simulink model "twobit"  (R2016b)
settings: Solver=VariableStepAuto  StartTime=0.0  StopTime=1024  RelTol=1e-3
libraries: xbsIndex_r4 x150, casper_library_misc x3, xps_library x1
settings Model: Creator=nivek  LastModifiedBy=nivek

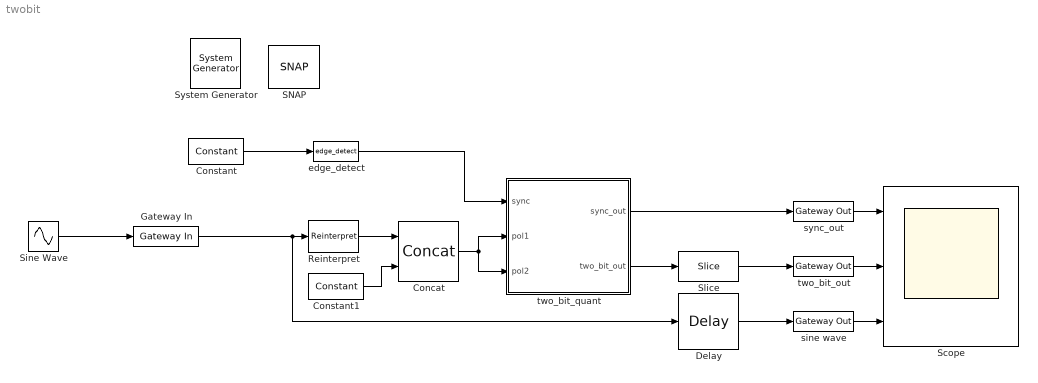
== system twobit ==
  " System Generator" : xbsIndex_r4/ System Generator  Tag=genX  xilinxfamily=kintex7  part=xc7k325t  speed=-3  package=fbg676  synthesis_tool=Vivado  clock_wrapper=Clock Enables  directory=./netlist  proj_type=Vivado  Synth_file=Vivado Synthesis Defaults  Impl_file=Vivado Implementation Defaults  testbench=off  simulink_period=1  sysclk_period=10  dcm_input_clock_period=10  incr_netlist=off  trim_vbits=Everywhere in SubSystem  dbl_ovrd=According to Block Masks  core_generation=According to Block Masks  run_coregen=off  deprecated_control=off  eval_field=0  block_type=sysgen
  Concat : xbsIndex_r4/Concat  num_inputs=2  dbl_ovrd=off  block_type=concat
  Constant : xbsIndex_r4/Constant  const=1.0  gui_display_data_type=Boolean  arith_type=Boolean  n_bits=16  bin_pt=14  preci_type=Single  exp_width=8  frac_width=24  explicit_period=on  period=1  equ=P=C  opselect=C  inp2=PCIN>>17  opr=+  inp1=P  carry=CIN  dbl_ovrd=off  block_type=constant
  Constant1 : xbsIndex_r4/Constant  const=0  gui_display_data_type=Fixed-point  arith_type=Unsigned  n_bits=18  bin_pt=0  preci_type=Single  exp_width=8  frac_width=24  explicit_period=on  period=1  equ=P=C  opselect=C  inp2=PCIN>>17  opr=+  inp1=P  carry=CIN  dbl_ovrd=off  block_type=constant
  Delay : xbsIndex_r4/Delay  rst=off  infoeditControl=Selection of Reset will increase slice count due to use of real FFs and instead of SRLs  en=off  latency=9  reg_retiming=off  dbl_ovrd=off  block_type=delay
  Gateway In : xbsIndex_r4/Gateway In  gui_display_data_type=Fixed-point  arith_type="Signed  (2's comp)"  n_bits=18  bin_pt=17  preci_type=Single  exp_width=8  frac_width=24  rows=1  columns=1  quantization="Round  (unbiased: +/- Inf)"  overflow=Saturate  period=1  UseAsADC=off  ADCChannel='1'  interface=None  automatic_assignment=on  address_offset=hex2dec('00')  intf_name=''  intf_description=''  default_value=0  timing_constraint=None  locs_specified=off  LOCs={}  io_standard={}  inherit_from_input=off  hdl_port=on  dbl_ovrd=off  block_type=gatewayin
  Reinterpret : xbsIndex_r4/Reinterpret  force_arith_type=on  arith_type=Unsigned  force_bin_pt=on  bin_pt=0  block_type=reinterpret
  SNAP : xps_library/Platforms/SNAP  Tag=xps:xsg  hw_sys=SNAP:xc7k160t  clk_src=adc0_clk  clk_rate=250  use_microblaze=off  sample_period=1  synthesis_tool=XST
  Scope : Scope  NumInputPorts=3
  Sine Wave : Sin  SineType=Sample based  Amplitude=0.875  Samples=128  SampleTime=1
  Slice : xbsIndex_r4/Slice  nbits=2  boolean_output=off  mode=Upper Bit Location + Width  bit1=0  base1=MSB of Input  bit0=0  base0=LSB of Input  dbl_ovrd=off  block_type=slice
  edge_detect : casper_library_misc/edge_detect  edge=Rising  polarity=Active High  x_in=[0 0.08 0.08 0.16 0.16 0.24 0.24 0.32 0.32 0.4]  y_in="[-1 -1  1  1  1  1  1  1  1  1]"  x_out=[0.6 0.68 0.68 0.76 0.76 0.84 0.84 0.92 0.92 1]  y_out="[-1 -1  1  1 -1 -1 -1 -1 -1 -1]"
  sine wave : xbsIndex_r4/Gateway Out  inherit_from_input=off  hdl_port=on  rows=1  columns=1  UseAsDAC=off  DACChannel='1'  interface=None  automatic_assignment=on  address_offset=hex2dec('00')  intf_name=''  intf_description=''  timing_constraint=None  locs_specified=off  LOCs={}  io_standard={}  block_type=gatewayout
  sync_out : xbsIndex_r4/Gateway Out  inherit_from_input=off  hdl_port=on  rows=1  columns=1  UseAsDAC=off  DACChannel='1'  interface=None  automatic_assignment=on  address_offset=hex2dec('00')  intf_name=''  intf_description=''  timing_constraint=None  locs_specified=off  LOCs={}  io_standard={}  block_type=gatewayout
  two_bit_out : xbsIndex_r4/Gateway Out  inherit_from_input=off  hdl_port=on  rows=1  columns=1  UseAsDAC=off  DACChannel='1'  interface=None  automatic_assignment=on  address_offset=hex2dec('00')  intf_name=''  intf_description=''  timing_constraint=None  locs_specified=off  LOCs={}  io_standard={}  block_type=gatewayout
  two_bit_quant : Subsystem
  wires:
  two_bit_out/1 -> Scope/2
  sync_out/1 -> Scope/1
  two_bit_quant/1(sync_out) -> sync_out/1
  two_bit_quant/2(two_bit_out) -> Slice/1
  Slice/1 -> two_bit_out/1
  edge_detect/1 -> two_bit_quant/1(sync)
  Constant/1 -> edge_detect/1
  Sine Wave/1 -> Gateway In/1
  sine wave/1 -> Scope/3
  Constant1/1 -> Concat/2
  Concat/1 -> two_bit_quant/3(pol2), two_bit_quant/2(pol1)
  Reinterpret/1 -> Concat/1
  Gateway In/1 -> Delay/1, Reinterpret/1
  Delay/1 -> sine wave/1

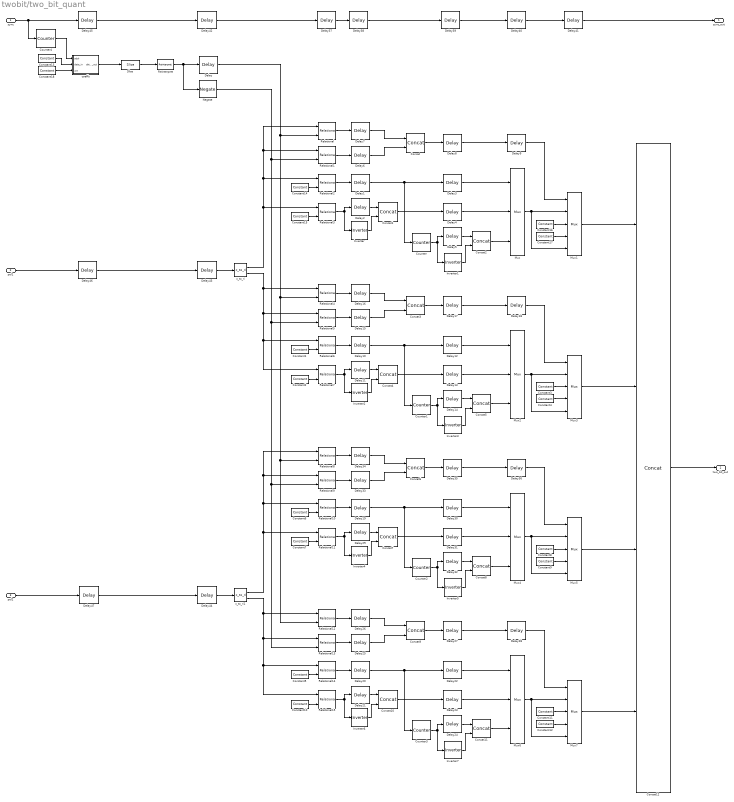
== system twobit/two_bit_quant ==
  sync : Inport
  pol1 : Inport  Port=2
  pol2 : Inport  Port=3
  Concat{,1..11} (12 alike) : xbsIndex_r4/Concat  num_inputs=2  dbl_ovrd=off  block_type=concat
  Concat12 : xbsIndex_r4/Concat  num_inputs=4  dbl_ovrd=off  block_type=concat
  Constant{1..2,5..7,10,14..15} (8 alike) : xbsIndex_r4/Constant  const=0  gui_display_data_type=Fixed-point  arith_type=Signed (2's comp)  n_bits=16  bin_pt=14  preci_type=Single  exp_width=8  frac_width=24  explicit_period=on  period=1  equ=P=C  opselect=C  inp2=PCIN>>17  opr=+  inp1=P  carry=CIN  dbl_ovrd=off  block_type=constant
  Constant{3,8,11,16} (4 alike) : xbsIndex_r4/Constant  const=0  gui_display_data_type=Fixed-point  arith_type=Unsigned  n_bits=2  bin_pt=0  preci_type=Single  exp_width=8  frac_width=24  explicit_period=on  period=1  equ=P=C  opselect=C  inp2=PCIN>>17  opr=+  inp1=P  carry=CIN  dbl_ovrd=off  block_type=constant
  Constant{4,9,12,17} (4 alike) : xbsIndex_r4/Constant  const=3  gui_display_data_type=Fixed-point  arith_type=Unsigned  n_bits=2  bin_pt=0  preci_type=Single  exp_width=8  frac_width=24  explicit_period=on  period=1  equ=P=C  opselect=C  inp2=PCIN>>17  opr=+  inp1=P  carry=CIN  dbl_ovrd=off  block_type=constant
  Constant13 : xbsIndex_r4/Constant  const=0  gui_display_data_type=Fixed-point  arith_type=Signed (2's comp)  n_bits=32  bin_pt=17  preci_type=Single  exp_width=8  frac_width=24  explicit_period=on  period=1  equ=P=C  opselect=C  inp2=PCIN>>17  opr=+  inp1=P  carry=CIN  dbl_ovrd=off  block_type=constant
  Constant18 : xbsIndex_r4/Constant  const=0  gui_display_data_type=Boolean  arith_type=Boolean  n_bits=16  bin_pt=14  preci_type=Single  exp_width=8  frac_width=24  explicit_period=on  period=1  equ=P=C  opselect=C  inp2=PCIN>>17  opr=+  inp1=P  carry=CIN  dbl_ovrd=off  block_type=constant
  Counter{,1..3} (4 alike) : xbsIndex_r4/Counter  cnt_type=Free Running  cnt_to=Inf  operation=Up  start_count=0  cnt_by_val=1  arith_type=Unsigned  n_bits=1  bin_pt=0  load_pin=off  rst=off  en=on  explicit_period=on  period=1  use_behavioral_HDL=off  implementation=Fabric  dbl_ovrd=off  block_type=counter
  Counter4 : xbsIndex_r4/Counter  cnt_type=Free Running  cnt_to=50  operation=Up  start_count=0  cnt_by_val=1  arith_type=Unsigned  n_bits=11  bin_pt=0  load_pin=off  rst=on  en=off  explicit_period=on  period=1  use_behavioral_HDL=off  implementation=Fabric  dbl_ovrd=off  block_type=counter
  Delay{,1..44} (45 alike) : xbsIndex_r4/Delay  rst=off  infoeditControl=Selection of Reset will increase slice count due to use of real FFs and instead of SRLs  en=off  latency=1  reg_retiming=off  dbl_ovrd=off  block_type=delay
  Delay45 : xbsIndex_r4/Delay  rst=off  infoeditControl=Selection of Reset will increase slice count due to use of real FFs and instead of SRLs  en=off  latency=3  reg_retiming=off  dbl_ovrd=off  block_type=delay
  Delay46 : xbsIndex_r4/Delay  rst=off  infoeditControl=Selection of Reset will increase slice count due to use of real FFs and instead of SRLs  en=off  latency=3  reg_retiming=off  dbl_ovrd=off  block_type=delay
  Delay47 : xbsIndex_r4/Delay  rst=off  infoeditControl=Selection of Reset will increase slice count due to use of real FFs and instead of SRLs  en=off  latency=3  reg_retiming=off  dbl_ovrd=off  block_type=delay
  Inverter{,1..7} (8 alike) : xbsIndex_r4/Inverter  en=off  latency=1  dbl_ovrd=off  block_type=inv
  Mux{,2,4,6} (4 alike) : xbsIndex_r4/Mux  inputs=2  en=off  latency=1  precision=Full  arith_type=Unsigned  n_bits=16  bin_pt=14  quantization=Truncate  overflow=Wrap  dbl_ovrd=off  block_type=mux
  Mux{1,3,5,7} (4 alike) : xbsIndex_r4/Mux  inputs=4  en=off  latency=1  precision=Full  arith_type=Unsigned  n_bits=16  bin_pt=14  quantization=Truncate  overflow=Wrap  dbl_ovrd=off  block_type=mux
  Negate : xbsIndex_r4/Negate  precision=User Defined  arith_type="Signed  (2's comp)"  n_bits=18  bin_pt=17  quantization=Truncate  overflow=Wrap  en=off  latency=1  dbl_ovrd=off  block_type=negate
  Reinterpret : xbsIndex_r4/Reinterpret  force_arith_type=on  arith_type="Signed  (2's comp)"  force_bin_pt=on  bin_pt=17  block_type=reinterpret
  Relational{,4,8,12} (4 alike) : xbsIndex_r4/Relational  mode=a>=b  op_type=Bool  en=off  latency=1  dbl_ovrd=off  block_type=relational
  Relational{1,5,9,13} (4 alike) : xbsIndex_r4/Relational  mode=a<=b  op_type=Bool  en=off  latency=1  dbl_ovrd=off  block_type=relational
  Relational{2,6,10,14} (4 alike) : xbsIndex_r4/Relational  mode=a=b  op_type=Bool  en=off  latency=1  dbl_ovrd=off  block_type=relational
  Relational{3,7,11,15} (4 alike) : xbsIndex_r4/Relational  mode=a>b  op_type=Bool  en=off  latency=1  dbl_ovrd=off  block_type=relational
  Slice : xbsIndex_r4/Slice  nbits=18  boolean_output=off  mode=Lower Bit Location + Width  bit1=0  base1=MSB of Input  bit0=0  base0=LSB of Input  dbl_ovrd=off  block_type=slice
  c_to_ri : casper_library_misc/c_to_ri  n_bits=18  bin_pt=17
  c_to_ri1 : casper_library_misc/c_to_ri  n_bits=18  bin_pt=17
  coeffs : Subsystem  Tag=xps:bram  AncestorBlock=xps_library/Memory/shared_bram  mask{arith_type=Unsigned, addr_width=11, data_width=32, reg_prim_output=on, reg_core_output=on, optimization=Minimum_Area, data_bin_pt=0, init_vals=ones(1, 2^11)*65536, sample_rate=1}
      mask prompts: arith_type "Output Data Type"; addr_width "Address width"; data_width "Data Width"; reg_prim_output "Register Primitive Output"; reg_core_output "Register Core Output"; data_bin_pt "Data Binary Point"; init_vals "Initial values (simulation only)"; sample_rate "Sample rate"
      mask init:
      | shared_bram_mask;
      mask TypeOptions arith_type: Unsigned | Signed  (2's comp)
      mask TypeOptions data_width: 8 | 16 | 32 | 64 | 128
      mask TypeOptions optimization: Minimum_Area | Low_Power
  sync_out : Outport
  two_bit_out : Outport  Port=2
  wires:
  Delay41/1 -> sync_out/1
  Delay37/1 -> Delay38/1
  Relational3/1 -> Delay2/1, Inverter/1
  Mux1/1 -> Concat12/1
  Delay5/1 -> Concat2/1
  Constant14/1 -> Relational2/2
  Constant16/1 -> Mux1/3
  Delay38/1 -> Delay39/1
  Delay3/1 -> Mux/1
  Concat2/1 -> Mux/3
  Delay9/1 -> Mux1/1
  Delay8/1 -> Delay9/1
  pol1/1 -> Delay46/1
  sync/1 -> Counter4/1, Delay45/1
  c_to_ri/1 -> Relational3/1, Relational2/1, Relational1/1, Relational/1
  Mux5/1 -> Concat12/3
  Constant15/1 -> Relational3/2
  Delay39/1 -> Delay40/1
  Delay6/1 -> Concat/2
  Mux7/1 -> Concat12/4
  Concat/1 -> Delay8/1
  Delay7/1 -> Concat/1
  Mux/1 -> Mux1/5, Mux1/2
  Inverter/1 -> Concat1/2
  Relational2/1 -> Delay1/1
  Concat12/1 -> two_bit_out/1
  Delay2/1 -> Concat1/1
  Delay1/1 -> Delay3/1, Counter/1
  Delay40/1 -> Delay41/1
  Delay4/1 -> Mux/2
  Relational1/1 -> Delay6/1
  Concat1/1 -> Delay4/1
  Mux3/1 -> Concat12/2
  Relational/1 -> Delay7/1
  Counter/1 -> Inverter1/1, Delay5/1
  Inverter1/1 -> Concat2/2
  Constant17/1 -> Mux1/4
  coeffs/1(data_out) -> Slice/1
  pol2/1 -> Delay47/1
  Delay42/1 -> Delay37/1
  Relational7/1 -> Delay11/1, Inverter2/1
  Delay14/1 -> Concat5/1
  Constant1/1 -> Relational6/2
  Constant3/1 -> Mux3/3
  Delay12/1 -> Mux2/1
  Concat5/1 -> Mux2/3
  Delay18/1 -> Mux3/1
  Delay17/1 -> Delay18/1
  c_to_ri/2 -> Relational7/1, Relational6/1, Relational5/1, Relational4/1
  Constant2/1 -> Relational7/2
  Delay15/1 -> Concat3/2
  Concat3/1 -> Delay17/1
  Delay16/1 -> Concat3/1
  Mux2/1 -> Mux3/5, Mux3/2
  Inverter2/1 -> Concat4/2
  Relational6/1 -> Delay10/1
  Delay11/1 -> Concat4/1
  Delay10/1 -> Delay12/1, Counter1/1
  Delay13/1 -> Mux2/2
  Relational5/1 -> Delay15/1
  Concat4/1 -> Delay13/1
  Relational4/1 -> Delay16/1
  Counter1/1 -> Inverter3/1, Delay14/1
  Inverter3/1 -> Concat5/2
  Constant4/1 -> Mux3/4
  Relational11/1 -> Inverter4/1, Delay29/1
  Delay32/1 -> Concat8/1
  Constant6/1 -> Relational10/2
  Constant8/1 -> Mux5/3
  Delay30/1 -> Mux4/1
  Concat8/1 -> Mux4/3
  Delay36/1 -> Mux5/1
  Delay35/1 -> Delay36/1
  c_to_ri1/1 -> Relational8/1, Relational9/1, Relational10/1, Relational11/1
  Constant7/1 -> Relational11/2
  Delay33/1 -> Concat6/2
  Concat6/1 -> Delay35/1
  Delay34/1 -> Concat6/1
  Mux4/1 -> Mux5/2, Mux5/5
  Inverter4/1 -> Concat7/2
  Relational10/1 -> Delay19/1
  Delay29/1 -> Concat7/1
  Delay19/1 -> Counter2/1, Delay30/1
  Delay31/1 -> Mux4/2
  Relational9/1 -> Delay33/1
  Concat7/1 -> Delay31/1
  Relational8/1 -> Delay34/1
  Counter2/1 -> Delay32/1, Inverter5/1
  Inverter5/1 -> Concat8/2
  Constant9/1 -> Mux5/4
  Relational15/1 -> Inverter6/1, Delay21/1
  Delay24/1 -> Concat11/1
  Constant5/1 -> Relational14/2
  Constant11/1 -> Mux7/3
  Delay22/1 -> Mux6/1
  Concat11/1 -> Mux6/3
  Delay28/1 -> Mux7/1
  Delay27/1 -> Delay28/1
  c_to_ri1/2 -> Relational12/1, Relational13/1, Relational14/1, Relational15/1
  Negate/1 -> Relational1/2, Relational5/2, Relational9/2, Relational13/2
  Constant10/1 -> Relational15/2
  Delay25/1 -> Concat9/2
  Concat9/1 -> Delay27/1
  Delay26/1 -> Concat9/1
  Mux6/1 -> Mux7/2, Mux7/5
  Inverter6/1 -> Concat10/2
  Relational14/1 -> Delay20/1
  Delay/1 -> Relational/2, Relational4/2, Relational12/2, Relational8/2
  Delay21/1 -> Concat10/1
  Delay20/1 -> Counter3/1, Delay22/1
  Delay23/1 -> Mux6/2
  Relational13/1 -> Delay25/1
  Concat10/1 -> Delay23/1
  Relational12/1 -> Delay26/1
  Counter3/1 -> Delay24/1, Inverter7/1
  Inverter7/1 -> Concat11/2
  Constant12/1 -> Mux7/4
  Delay43/1 -> c_to_ri/1
  Delay44/1 -> c_to_ri1/1
  Constant18/1 -> coeffs/3(we)
  Constant13/1 -> coeffs/2(data_in)
  Counter4/1 -> coeffs/1(addr)
  Delay45/1 -> Delay42/1
  Delay46/1 -> Delay43/1
  Delay47/1 -> Delay44/1
  Slice/1 -> Reinterpret/1
  Reinterpret/1 -> Delay/1, Negate/1

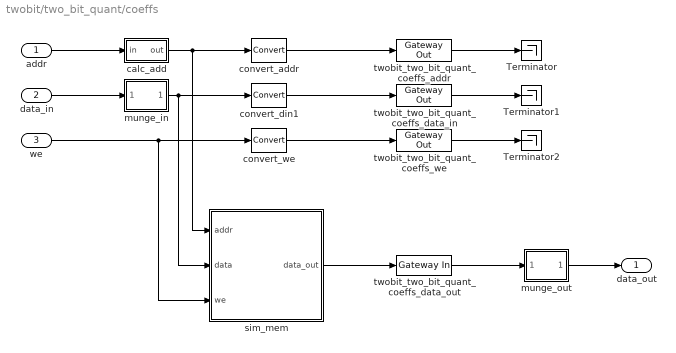
== system twobit/two_bit_quant/coeffs ==
  addr : Inport
  data_in : Inport  Port=2
  we : Inport  Port=3
  Terminator : Terminator
  Terminator1 : Terminator
  Terminator2 : Terminator
  calc_add : Subsystem  mask{data_width=32, addr_width=11, sample_rate=sample_rate}
      mask prompts: data_width "data width"; addr_width "address width"; sample_rate "sample rate"
  convert_addr : xbsIndex_r4/Convert  gui_display_data_type=Fixed-point  arith_type=Unsigned  n_bits=addr_width  bin_pt=0  float_type=Single  exp_bits=8  fraction_bits=24  quantization=Truncate  overflow=Wrap  en=off  latency=0  pipeline=off  dbl_ovrd=off  block_type=convert
      settings: xl_area=[0, 0, 0, 0, 0, 0, 0]
  convert_din1 : xbsIndex_r4/Convert  gui_display_data_type=Fixed-point  arith_type=Unsigned  n_bits=32  bin_pt=0  float_type=Single  exp_bits=8  fraction_bits=24  quantization=Truncate  overflow=Wrap  en=off  latency=0  pipeline=off  dbl_ovrd=off  block_type=convert
      settings: xl_area=[0, 0, 0, 0, 0, 0, 0]
  convert_we : xbsIndex_r4/Convert  gui_display_data_type=Fixed-point  arith_type=Unsigned  n_bits=1  bin_pt=0  float_type=Single  exp_bits=8  fraction_bits=24  quantization=Truncate  overflow=Wrap  en=off  latency=0  pipeline=off  dbl_ovrd=off  block_type=convert
      settings: xl_area=[0, 0, 0, 0, 0, 0, 0]
  munge_in : Subsystem  AncestorBlock=casper_library_flow_control/munge  mask(munge){divisions=1, div_size=32, order=[0], arith_type_out=Unsigned, bin_pt_out=0}
      mask prompts: divisions "Number of divisions"; div_size "Division size (bits)"; order "Division packing order"; arith_type_out "Output arithmetic type"; bin_pt_out "Output binary point"
      mask help: Splits an input bus into the specified number of divisions and then recombines them in the order specified (most significant division = 0,least = number divisions-1)
      mask init:
      | munge_init(gcb, ...
      |     'divisions', divisions, ...
      |     'div_size', div_size, ...
      |     'order', order, ...
      |     'arith_type_out', arith_type_out, ...
      |     'bin_pt_out', bin_pt_out);
      settings: AttributesFormatString=|
      | split:32
      | join:0
      | Unsigned [32,0]
      mask TypeOptions arith_type_out: Unsigned | Signed  (2's comp) | Floating-point
  munge_out : Subsystem  AncestorBlock=casper_library_flow_control/munge  mask(munge){divisions=1, div_size=32, order=[0], arith_type_out=Unsigned, bin_pt_out=0}
      mask prompts: divisions "Number of divisions"; div_size "Division size (bits)"; order "Division packing order"; arith_type_out "Output arithmetic type"; bin_pt_out "Output binary point"
      mask help: Splits an input bus into the specified number of divisions and then recombines them in the order specified (most significant division = 0,least = number divisions-1)
      mask init:
      | munge_init(gcb, ...
      |     'divisions', divisions, ...
      |     'div_size', div_size, ...
      |     'order', order, ...
      |     'arith_type_out', arith_type_out, ...
      |     'bin_pt_out', bin_pt_out);
      settings: AttributesFormatString=|
      | split:32
      | join:0
      | Unsigned [32,0]
      mask TypeOptions arith_type_out: Unsigned | Signed  (2's comp) | Floating-point
  sim_mem : Subsystem  mask{arith_type=Unsigned, addr_width=11, data_width=32, data_bin_pt=0, init_vals=[65536  65536  65536  65536  65536  65536  65536  65536  65536  65536  65536  65536  65536  65536  65536  65536  65536  65536  65536  65536  65536  65536  65536  65536  65536  65536  65536  65536  65536  65536  65536  65536  65536  65536  65536  65536  65536  65536  65536  65536  65536  65536  65536  65536  65536  65536  65536  65536  65536  65536  65536  65536  65536  65536  65536  65536  65536  65536  65536  65536  65536  65536  65536  65536  65536  65536  65536  65536  65536  65536  65536  65536  65536  65536  65536  65536  65536  65536  65536  65536  65536  65536  65536  65536  65536  65536  65536  65536  65536  65536  65536  65536  65536  65536  65536  65536  65536  65536  65536  65536  65536  65536  65536  65536  65536  65536  65536  65536  65536  65536  65536  65536  65536  65536  65536  65536  65536  65536  65536  65536  65536  65536  65536  65536  65536  65536  65536  65536  65536  65536  65536  65536  65536  65536  65536  65536  65536  65536  65536  65536  65536  65536  65536  65536  65536  65536  65536  65536  65536  65536  65536  65536  65536  65536  65536  65536  65536  65536  65536  65536  65536  65536  65536  65536  65536  65536  65536  65536  65536  65536  65536  65536  65536  65536  65536  65536  65536  65536  65536  65536  65536  65536  65536  65536  65536  65536  65536  65536  65536  65536  65536  65536  65536  65536  65536  65536  65536  65536  65536  65536  65536  65536  65536  65536  65536  65536  65536  65536  65536  65536  65536  65536  65536  65536  65536  65536  65536  65536  65536  65536  65536  65536  65536  65536  65536  65536  65536  65536  65536  65536  65536  65536  65536  65536  65536  65536  65536  65536  65536  65536  65536  65536  65536  65536  65536  65536  65536  65536  65536  65536  65536  65536  65536  65536  65536  65536  65536  65536  65536  65536  65536  65536  65536  65536  65536  65536  65536  65536  65536  65536  65536  65536  65536  65536  65536  65536  65536  65536  65536  65536  65536  65536  65536  65536  65536  65536  65536  65536  65536  65536  65536  65536  65536  65536  65536  65536  65536  65536  65536  65536  65536  65536  65536  65536  65536  65536  65536  65536  65536  65536  65536  65536  65536  65536  65536  65536  65536  65536  65536  65536  65536  65536  65536  65536  65536  65536  65536  65536  65536  65536  65536  65536  65536  65536  65536  65536  65536  65536  65536  65536  65536  65536  65536  65536  65536  65536  65536  65536  65536  65536  65536  65536  65536  65536  65536  65536  65536  65536  65536  65536  65536  65536  65536  65536  65536  65536  65536  65536  65536  65536  65536  65536  65536  65536  65536  65536  65536  65536  65536  65536  65536  65536  65536  65536  65536  65536  65536  65536  65536  65536  65536  65536  65536  65536  65536  65536  65536  65536  65536  65536  65536  65536  65536  65536  65536  65536  65536  65536  65536  65536  65536  65536  65536  65536  65536  65536  65536  65536  65536  65536  65536  65536  65536  65536  65536  65536  65536  65536  65536  65536  65536  65536  65536  65536  65536  65536  65536  65536  65536  65536  65536  65536  65536  65536  65536  65536  65536  65536  65536  65536  65536  65536  65536  65536  65536  65536  65536  65536  65536  65536  65536  65536  65536  65536  65536  65536  65536  65536  65536  65536  65536  65536  65536  65536  65536  65536  65536  65536  65536  65536  65536  65536  65536  65536  65536  65536  65536  65536  65536  65536  65536  65536  65536  65536  65536  65536  65536  65536  65536  65536  65536  65536  65536  65536  65536  65536  65536  65536  65536  65536  65536  65536  65536  65536  65536  65536  65536  65536  65536  65536  65536  65536  65536  65536  65536  65536  65536  65536  65536  65536  65536  65536  65536  65536  65536  65536  65536  65536  65536  65536  65536  65536  65536  65536  65536  65536  65536  65536  65536  65536  65536  65536  65536  65536  65536  65536  65536  65536  65536  65536  65536  65536  65536  65536  65536  65536  65536  65536  65536  65536  65536 ...(+10338 chars)], sample_rate=1, latency=3}
      mask prompts: arith_type "Output Data Type"; addr_width "Address width"; data_width "Data width"; data_bin_pt "Data Binary Point"; init_vals "Initial values"; sample_rate "Sample rate"
      mask init:
      | % set_param([gcb, '/data_to_xilinx'], 'arith_type', arith_type)
      | % set_param([gcb, '/data_to_xilinx'], 'n_bits', get_param(gcb, 'data_width'))
      mask TypeOptions arith_type: Unsigned | Signed  (2's comp)
      mask TypeOptions data_width: 8 | 16 | 32 | 64 | 128
  twobit_two_bit_quant_coeffs_addr : xbsIndex_r4/Gateway Out  inherit_from_input=off  hdl_port=on  rows=1  columns=1  UseAsDAC=off  DACChannel='1'  interface=None  automatic_assignment=on  address_offset=hex2dec('00')  intf_name=''  intf_description=''  timing_constraint=None  locs_specified=off  LOCs={'A5','B9','A9','C1','A3','G6','E9','A6','A7','A8','B8','B1','B3','D9','B5','B4','B6','C2'}  io_standard={}  block_type=gatewayout
      settings: infoedit="Gateway out block.  Converts Xilinx fixed point inputs into ouputs of type Simulink integer, double, or fixed point.<P><P>Hardware notes:  In hardware these blocks become top level output ports or are discarded, depending on how they are configured."  sginterface={'Nallatech'=>{'xdspkit'=>{'non_memory_mapped_port'=>'uprev_Shared_BRAM_addr'}},'Xilinx'=>{'jtaghwcosim'=>{'non_memory_mapped_port'=>'uprev_Shared_BRAM_addr'},'xdspkit'=>{'non_memory_mapped_port'=>'uprev_Shared_BRAM_addr'}}}  xl_area=[0, 0, 0, 0, 0, 0, 0]
  twobit_two_bit_quant_coeffs_data_in : xbsIndex_r4/Gateway Out  inherit_from_input=off  hdl_port=on  rows=1  columns=1  UseAsDAC=off  DACChannel='1'  interface=None  automatic_assignment=on  address_offset=hex2dec('00')  intf_name=''  intf_description=''  timing_constraint=None  locs_specified=off  LOCs={'B21','B22','A22','B23','B19','C19','A20','A21','A23','B24','A24','A25','E18','D18','C18','B18'}  io_standard={}  block_type=gatewayout
      settings: infoedit="Gateway out block.  Converts Xilinx fixed point inputs into ouputs of type Simulink integer, double, or fixed point.<P><P>Hardware notes:  In hardware these blocks become top level output ports or are discarded, depending on how they are configured."  sginterface={'Nallatech'=>{'xdspkit'=>{'non_memory_mapped_port'=>'uprev_Shared_BRAM_data_in'}},'Xilinx'=>{'jtaghwcosim'=>{'non_memory_mapped_port'=>'uprev_Shared_BRAM_data_in'},'xdspkit'=>{'non_memory_mapped_port'=>'uprev_Shared_BRAM_data_in'}}}  xl_area=[0, 0, 0, 0, 0, 0, 0]
  twobit_two_bit_quant_coeffs_data_out : xbsIndex_r4/Gateway In  gui_display_data_type=Fixed-point  arith_type=Unsigned  n_bits=32  bin_pt=0  preci_type=Single  exp_width=8  frac_width=24  rows=1  columns=1  quantization=Truncate  overflow=Wrap  period=sample_rate  UseAsADC=off  ADCChannel='1'  interface=None  automatic_assignment=on  address_offset=hex2dec('00')  intf_name=''  intf_description=''  default_value=0  timing_constraint=None  locs_specified=off  LOCs={}  io_standard={}  inherit_from_input=off  hdl_port=on  dbl_ovrd=off  block_type=gatewayin
      settings: xl_area=[0, 0, 0, 0, 0, 0, 0]
  twobit_two_bit_quant_coeffs_we : xbsIndex_r4/Gateway Out  inherit_from_input=off  hdl_port=on  rows=1  columns=1  UseAsDAC=off  DACChannel='1'  interface=None  automatic_assignment=on  address_offset=hex2dec('00')  intf_name=''  intf_description=''  timing_constraint=None  locs_specified=off  LOCs={'A14'}  io_standard={}  block_type=gatewayout
      settings: infoedit="Gateway out block.  Converts Xilinx fixed point inputs into ouputs of type Simulink integer, double, or fixed point.<P><P>Hardware notes:  In hardware these blocks become top level output ports or are discarded, depending on how they are configured."  xl_area=[0, 0, 0, 0, 0, 0, 0]
  data_out : Outport
  wires:
  munge_out/1(dout) -> data_out/1
  sim_mem/1(data_out) -> twobit_two_bit_quant_coeffs_data_out/1
  twobit_two_bit_quant_coeffs_data_out/1 -> munge_out/1(din)
  convert_addr/1 -> twobit_two_bit_quant_coeffs_addr/1
  convert_din1/1 -> twobit_two_bit_quant_coeffs_data_in/1
  data_in/1 -> munge_in/1(din)
  calc_add/1(out) -> sim_mem/1(addr), convert_addr/1
  twobit_two_bit_quant_coeffs_we/1 -> Terminator2/1
  twobit_two_bit_quant_coeffs_data_in/1 -> Terminator1/1
  twobit_two_bit_quant_coeffs_addr/1 -> Terminator/1
  convert_we/1 -> twobit_two_bit_quant_coeffs_we/1
  addr/1 -> calc_add/1(in)
  we/1 -> sim_mem/3(we), convert_we/1
  munge_in/1(dout) -> sim_mem/2(data), convert_din1/1

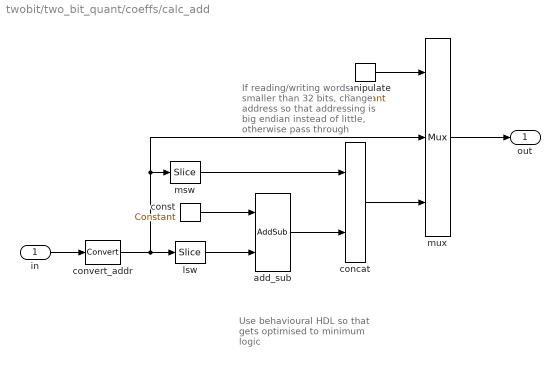
== system twobit/two_bit_quant/coeffs/calc_add ==
  note: Use behavioural HDL
      | so that gets optimised
      | to minimum logic
  note: If reading/writing words
      | smaller than 32 bits,
      | change address so
      | that addressing is
      | big endian instead of
      | little, otherwise
      | pass through
  in : Inport
  add_sub : xbsIndex_r4/AddSub  mode=Subtraction  use_carryin=off  use_carryout=off  en=off  latency=0  precision=User Defined  arith_type=Unsigned  n_bits=max(1, log2(32/data_width))  bin_pt=0  quantization=Truncate  overflow=Wrap  use_behavioral_HDL=on  hw_selection=Fabric  pipelined=off  dbl_ovrd=off  block_type=addsub
  concat : xbsIndex_r4/Concat  num_inputs=2  dbl_ovrd=off  block_type=concat
  const : xbsIndex_r4/Constant  const=max(0, 32/data_width-1)  gui_display_data_type=Fixed-point  arith_type=Unsigned  n_bits=max(1, log2(32/data_width))  bin_pt=0  preci_type=Single  exp_width=8  frac_width=24  explicit_period=on  period=sample_rate  equ=P=C  opselect=C  inp2=PCIN>>17  opr=+  inp1=P  carry=CIN  dbl_ovrd=off  block_type=constant
      settings: block_version=11.4
  convert_addr : xbsIndex_r4/Convert  gui_display_data_type=Fixed-point  arith_type=Unsigned  n_bits=addr_width  bin_pt=0  float_type=Single  exp_bits=8  fraction_bits=24  quantization=Truncate  overflow=Wrap  en=off  latency=0  pipeline=off  dbl_ovrd=off  block_type=convert
      settings: xl_area=[0, 0, 0, 0, 0, 0, 0]
  lsw : xbsIndex_r4/Slice  nbits=max(1, log2(32/data_width))  boolean_output=off  mode=Lower Bit Location + Width  bit1=0  base1=MSB of Input  bit0=0  base0=LSB of Input  dbl_ovrd=off  block_type=slice
  manipulate : xbsIndex_r4/Constant  const=min(1, floor(32/data_width) - 1)  gui_display_data_type=Fixed-point  arith_type=Unsigned  n_bits=1  bin_pt=0  preci_type=Single  exp_width=8  frac_width=24  explicit_period=on  period=sample_rate  equ=P=C  opselect=C  inp2=PCIN>>17  opr=+  inp1=P  carry=CIN  dbl_ovrd=off  block_type=constant
      settings: block_version=11.4
  msw : xbsIndex_r4/Slice  nbits=addr_width - max(1, log2(32/data_width))  boolean_output=off  mode=Upper Bit Location + Width  bit1=0  base1=MSB of Input  bit0=0  base0=LSB of Input  dbl_ovrd=off  block_type=slice
  mux : xbsIndex_r4/Mux  inputs=2  en=off  latency=0  precision=Full  arith_type=Unsigned  n_bits=16  bin_pt=14  quantization=Truncate  overflow=Wrap  dbl_ovrd=off  block_type=mux
      settings: block_version=11.4
  out : Outport
  wires:
  convert_addr/1 -> mux/2, msw/1, lsw/1
  const/1 -> add_sub/1
  lsw/1 -> add_sub/2
  mux/1 -> out/1
  manipulate/1 -> mux/1
  concat/1 -> mux/3
  msw/1 -> concat/1
  add_sub/1 -> concat/2
  in/1 -> convert_addr/1

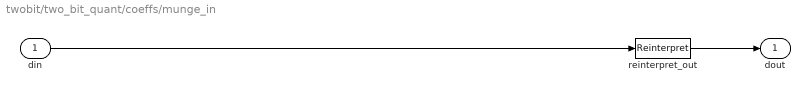
== system twobit/two_bit_quant/coeffs/munge_in ==
  din : Inport
  reinterpret_out : xbsIndex_r4/Reinterpret  force_arith_type=on  arith_type=Unsigned  force_bin_pt=on  bin_pt=0  block_type=reinterpret
  dout : Outport
  wires:
  reinterpret_out/1 -> dout/1
  din/1 -> reinterpret_out/1

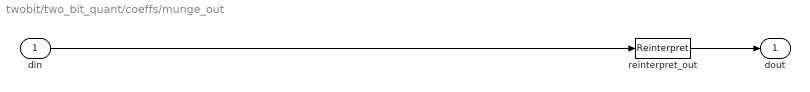
== system twobit/two_bit_quant/coeffs/munge_out ==
  din : Inport
  reinterpret_out : xbsIndex_r4/Reinterpret  force_arith_type=on  arith_type=Unsigned  force_bin_pt=on  bin_pt=0  block_type=reinterpret
  dout : Outport
  wires:
  reinterpret_out/1 -> dout/1
  din/1 -> reinterpret_out/1

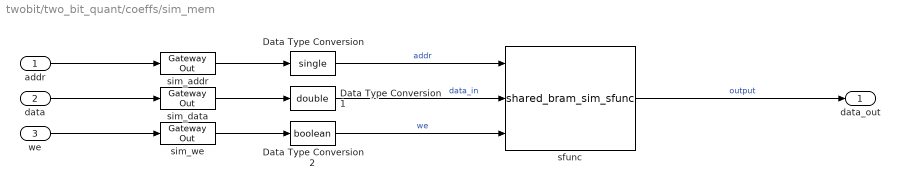
== system twobit/two_bit_quant/coeffs/sim_mem ==
  addr : Inport
  data : Inport  Port=2
  we : Inport  Port=3
  Data Type Conversion : DataTypeConversion  OutDataTypeStr=single
  Data Type Conversion1 : DataTypeConversion  OutDataTypeStr=double
  Data Type Conversion2 : DataTypeConversion  OutDataTypeStr=boolean
  sfunc : M-S-Function  FunctionName=shared_bram_sim_sfunc  Parameters=depth_bits, latency, init_vals  mask{depth_bits=addr_width, latency=latency, init_vals=init_vals}
      mask prompts: depth_bits "Depth (2^?):"; latency "Latency (>=1):"; init_vals "Initial values:"
      mask Callback latency:
      | latency = str2double(get_param(gcb, 'latency'));
      | if latency < 1
      |     errordlg('Cannot have latency less than one.');
      |     set_param(gcb, 'latency', '1');
      | end
  sim_addr : xbsIndex_r4/Gateway Out  inherit_from_input=off  hdl_port=off  rows=1  columns=1  UseAsDAC=off  DACChannel='1'  interface=None  automatic_assignment=on  address_offset=hex2dec('00')  intf_name=''  intf_description=''  timing_constraint=None  locs_specified=off  LOCs={}  io_standard={}  block_type=gatewayout
  sim_data : xbsIndex_r4/Gateway Out  inherit_from_input=off  hdl_port=off  rows=1  columns=1  UseAsDAC=off  DACChannel='1'  interface=None  automatic_assignment=on  address_offset=hex2dec('00')  intf_name=''  intf_description=''  timing_constraint=None  locs_specified=off  LOCs={}  io_standard={}  block_type=gatewayout
  sim_we : xbsIndex_r4/Gateway Out  inherit_from_input=off  hdl_port=off  rows=1  columns=1  UseAsDAC=off  DACChannel='1'  interface=None  automatic_assignment=on  address_offset=hex2dec('00')  intf_name=''  intf_description=''  timing_constraint=None  locs_specified=off  LOCs={}  io_standard={}  block_type=gatewayout
  data_out : Outport
  wires:
  sfunc/1 -> data_out/1  "output"
  Data Type Conversion2/1 -> sfunc/3  "we"
  Data Type Conversion1/1 -> sfunc/2  "data_in"
  Data Type Conversion/1 -> sfunc/1  "addr"
  sim_we/1 -> Data Type Conversion2/1
  sim_data/1 -> Data Type Conversion1/1
  sim_addr/1 -> Data Type Conversion/1
  we/1 -> sim_we/1
  data/1 -> sim_data/1
  addr/1 -> sim_addr/1
